simulink model "cm_test"  (R2015a)
settings: Solver=ode45  StartTime=0.0  StopTime=inf  MaxStep=1e-3  RelTol=1e-3
values from neighbouring files (symbols this model uses):
  ctr_law = struct    [Parameters.m]
  IMU = struct    [Parameters.m]
  lateral_control = true    [Parameters.m]
  longit_control = true    [Parameters.m]
  low_ctr = struct    [Parameters.m]
  mag = struct    [Parameters.m]
  steer_flag = 0    [Parameters.m]
  steer_sensor = struct    [Parameters.m]
  vhcl = struct    [Parameters.m]
undefined symbols (not defined in the file or in its folder): odo
libraries: CarMaker4SL x29, dspquant2 x6, simulink x1, aerolibtransform2 x1
(part 1 of 2)
settings Model: ExtModeAutoUpdateStatusClock=off  Creator=fh  LastModifiedBy=Robot
settings DataIOCC: SignalLoggingSaveFormat=ModelDataLogs  SignalLoggingName=sigsOut
settings OptimizationCC: BooleanDataType=off  ExpressionDepthLimit=2147483647  InitFltsAndDblsToZero=on
settings DebuggingCC: SaveWithParameterizedLinksMsg=none  SignalResolutionControl=TryResolveAllWithWarning  MultiTaskDSMMsg=warning  MultiTaskCondExecSysMsg=none  StateNameClashWarn=warning
settings HardwareCC: TargetUnknown=on
settings CodeAppCC: MaxIdLength=63
settings GRTTargetCC: TargetFcnLib=ansi_tfl_tmw.mat  CombineOutputUpdateFcns=off  GRTInterface=on
settings ConfigComp: CovMetricSettings=dw  CovHtmlReporting=on  CovSaveCumulativeToWorkspaceVar=on  CovSaveSingleToWorkspaceVar=on  CovExternalEMLEnable=off  CovSFcnEnable=off

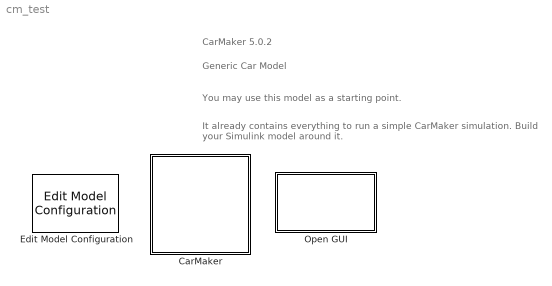
== system cm_test ==
  note: Generic Car Model
  note: You may use this model as a starting point.
  note: It already contains everything to run a simple CarMaker simulation.
      | Build your Simulink model around it.
  note: CarMaker 5.0.2
  CarMaker : Subsystem  TreatAsAtomicUnit=on
      mask Display: image(imread('CarMaker4SLss.bmp'));
  Edit Model Configuration : CarMaker4SL/Edit Model Configuration
  Open GUI : Subsystem  LoadFcn=if ~length(which('cmcmd')), cmenv; end
      settings: OpenFcn=cmblockmagic('gui_fix_display'); CM_Simulink
      mask Display: image(imread('CarMakerGUI.bmp'));

== system cm_test/CarMaker ==
  CM_FIRST : Subsystem
  CM_LAST : Subsystem
  DrivMan : Subsystem
  Ground : Ground
  IPG Vehicle : Subsystem  TreatAsAtomicUnit=on
  Terminator : Terminator
  VehicleControl : Subsystem
  wires:
  DrivMan/2(DrivMan.Out) -> VehicleControl/2(DrivMan.In)
  DrivMan/1(Sync_Out) -> VehicleControl/1(Sync_In)
  CM_FIRST/2(Env.Misc) -> DrivMan/2(Env.Misc)
  CM_FIRST/1(Sync_Out) -> DrivMan/1(Sync_In)
  CM_LAST/1(Sync_Out) -> Terminator/1
  IPG Vehicle/1(Sync_Out) -> CM_LAST/1(Sync_In)
  VehicleControl/1(Sync_Out) -> IPG Vehicle/1(Sync_In)
  VehicleControl/3(VhclCtrl.Steering) -> IPG Vehicle/3(VhclCtrl.Steering)
  VehicleControl/4(Vhcl.Wheel.In) -> IPG Vehicle/4(Vhcl.Wheel.In)
  VehicleControl/5(Vhcl.Misc) -> IPG Vehicle/5(Vhcl.Misc)
  VehicleControl/6(VhclCtrl.Brake) -> IPG Vehicle/6(VhclCtrl.Brake)
  VehicleControl/7(VhclCtrl.PT) -> IPG Vehicle/7(VhclCtrl.PT)
  VehicleControl/2(Vhcl.Model.Source) -> IPG Vehicle/2(Vhcl.Model.Source)
  Ground/1 -> CM_FIRST/1(Sync_In)

== system cm_test/Open GUI ==
  S-Function : S-Function  FunctionName=cm_gui

== system cm_test/CarMaker/CM_FIRST ==
  Sync_In : Inport
  Bus Creator1 : BusCreator  Inputs=9
  Demux : Demux  Outputs=9
  Environment : S-Function  FunctionName=CM_Sfun  Parameters='Environment'
  IoIn : S-Function  FunctionName=CM_Sfun  Parameters='IoIn'
  Sync_Out : Outport
  Env.Misc : Outport  Port=2
  wires:
  Bus Creator1/1 -> Env.Misc/1
  Environment/2 -> Demux/1
  Demux/4 -> Bus Creator1/4  "Env AirHumidity"
  Demux/3 -> Bus Creator1/3  "Env AirPressure"
  Demux/2 -> Bus Creator1/2  "Env AirDensity"
  Demux/1 -> Bus Creator1/1  "Env Temperature"
  Environment/1 -> Sync_Out/1
  IoIn/1 -> Environment/1
  Sync_In/1 -> IoIn/1
  Demux/5 -> Bus Creator1/5  "Env Time"
  Demux/6 -> Bus Creator1/6  "Env SolarRadiation"
  Demux/7 -> Bus Creator1/7  "Env WindVel_tot x"
  Demux/8 -> Bus Creator1/8  "Env WindVel_tot y"
  Demux/9 -> Bus Creator1/9  "Env WindVel_tot z"

== system cm_test/CarMaker/CM_LAST ==
  Sync_In : Inport
  CM_User : S-Function  FunctionName=CM_Sfun  Parameters='CM_User'
  IoOut : S-Function  FunctionName=CM_Sfun  Parameters='IoOut'
  Sync_Out : Outport
  wires:
  IoOut/1 -> Sync_Out/1
  CM_User/1 -> IoOut/1
  Sync_In/1 -> CM_User/1

== system cm_test/CarMaker/DrivMan ==
  note: There's rarely a reason to override DrivMan signals.
      | Use the VehicleControl interface for this purpose.
  Sync_In : Inport
  Env.Misc : Inport  Port=2
  BusCreator : BusCreator  Inputs=17
  Demux : Demux  Outputs=17
  DrivMan : S-Function  FunctionName=CM_Sfun  Parameters='DrivMan'
  Sync_Out : Outport
  DrivMan.Out : Outport  Port=2
  wires:
  Demux/17 -> BusCreator/17  "DrivMan Steering Trq"
  Demux/16 -> BusCreator/16  "DrivMan Steering AngAcc"
  Demux/15 -> BusCreator/15  "DrivMan Steering AngVel"
  Demux/14 -> BusCreator/14  "DrivMan Steering Ang"
  Demux/13 -> BusCreator/13  "DrivMan Gas"
  Demux/12 -> BusCreator/12  "DrivMan Clutch"
  Demux/11 -> BusCreator/11  "DrivMan BrakePark"
  Demux/10 -> BusCreator/10  "DrivMan Brake"
  Demux/9 -> BusCreator/9  "DrivMan GearNo"
  Demux/8 -> BusCreator/8  "DrivMan SelectorCtrl"
  Demux/7 -> BusCreator/7  "DrivMan UserSignal4"
  Demux/6 -> BusCreator/6  "DrivMan UserSignal3"
  Demux/5 -> BusCreator/5  "DrivMan UserSignal2"
  Demux/4 -> BusCreator/4  "DrivMan UserSignal1"
  Demux/3 -> BusCreator/3  "DrivMan UserSignal0"
  Demux/2 -> BusCreator/2  "DrivMan Key"
  Demux/1 -> BusCreator/1  "DrivMan SST"
  Env.Misc/1 -> DrivMan/2
  Sync_In/1 -> DrivMan/1
  DrivMan/1 -> Sync_Out/1
  BusCreator/1 -> DrivMan.Out/1
  DrivMan/2 -> Demux/1

== system cm_test/CarMaker/IPG Vehicle ==
  Sync_In : Inport
  Vhcl.Model.Source : Inport  Port=2
  VhclCtrl.Steering : Inport  Port=3
  Vhcl.Wheel.In : Inport  Port=4
  Vhcl.Misc : Inport  Port=5
  VhclCtrl.Brake : Inport  Port=6
  VhclCtrl.PT : Inport  Port=7
  Brake : Subsystem
  CarAndTrailer : Subsystem
  PowerTrain : Subsystem
  Stop Simulation : Stop
  VehicleSource_BuiltIn : simulink/Logic and Bit Operations/Compare To Constant  relop=~=  const=1  OutDataTypeStr=boolean  ZeroCross=off
  Sync_Out : Outport
  wires:
  VhclCtrl.PT/1 -> PowerTrain/3(VhclCtrl.PT)
  Brake/1(Sync_Out) -> PowerTrain/1(Sync_In)
  CarAndTrailer/1(Sync_Out) -> Brake/1(Sync_In)
  CarAndTrailer/2(Brake.IF.In) -> Brake/2(Brake.IF.In)
  VhclCtrl.Brake/1 -> Brake/3(VhclCtrl.Brake)
  PowerTrain/1(Sync_Out) -> Sync_Out/1
  Vhcl.Misc/1 -> CarAndTrailer/4(Vhcl.Misc)
  Vhcl.Wheel.In/1 -> CarAndTrailer/3(Vhcl.Wheel.In)
  VhclCtrl.Steering/1 -> CarAndTrailer/2(VhclCtrl.Steering)
  Sync_In/1 -> CarAndTrailer/1(Sync_In)
  Vhcl.Model.Source/1 -> VehicleSource_BuiltIn/1
  VehicleSource_BuiltIn/1 -> Stop Simulation/1
  Brake/2(Vhcl.Wheel.PT) -> PowerTrain/2(Vhcl.Wheel.PT)

== system cm_test/CarMaker/VehicleControl ==
  note: When implementing a vehicle control model,
      | be sure to add '-disablevehiclecontrol' to the command line arguments
      | in the CarMaker Model Configuration block.
      | Otherwise your model will possibly not see the original DrivMan signals
      | on its inputs, but those of a currently activated C-coded vehicle control model instead.
  Sync_In : Inport
  DrivMan.In : Inport  Port=2
  Autonomous driving : Subsystem
  Bus Creator2 : BusCreator  Inputs=2
  CreateBus Vhcl.Misc : Subsystem
  CreateBus Vhcl.Wheel.In : Subsystem
  CreateBus VhclCtrl : Subsystem
  CreateBus VhclCtrl.PT : Subsystem
  CreateBus VhclCtrl.Steering : Subsystem
  Demux2 : Demux  Outputs=2
  Sensors : Subsystem
  VehicleControl : S-Function  FunctionName=CM_Sfun  Parameters='VehicleControl'
  VehicleControlUpd : S-Function  FunctionName=CM_Sfun  Parameters='VehicleControlUpd'
  Sync_Out : Outport
  Vhcl.Model.Source : Outport  Port=2
  VhclCtrl.Steering : Outport  Port=3
  Vhcl.Wheel.In : Outport  Port=4
  Vhcl.Misc : Outport  Port=5
  VhclCtrl.Brake : Outport  Port=6
  VhclCtrl.PT : Outport  Port=7
  wires:
  VehicleControl/2 -> CreateBus VhclCtrl/1(Driver_In)
  VehicleControlUpd/2 -> Vhcl.Model.Source/1
  VehicleControlUpd/4 -> CreateBus Vhcl.Wheel.In/1(In1)
  VehicleControlUpd/5 -> CreateBus Vhcl.Misc/1(In1)
  VehicleControlUpd/6 -> Demux2/1
  VehicleControlUpd/7 -> CreateBus VhclCtrl.PT/1(In1)
  VehicleControlUpd/3 -> CreateBus VhclCtrl.Steering/1(In1)
  CreateBus Vhcl.Misc/1(Out1) -> Vhcl.Misc/1
  CreateBus Vhcl.Wheel.In/1(Out1) -> Vhcl.Wheel.In/1
  DrivMan.In/1 -> VehicleControl/2
  VehicleControl/1 -> VehicleControlUpd/1
  Sync_In/1 -> VehicleControl/1
  CreateBus VhclCtrl.PT/1(Out1) -> VhclCtrl.PT/1
  Bus Creator2/1 -> VhclCtrl.Brake/1
  CreateBus VhclCtrl.Steering/1(Out1) -> VhclCtrl.Steering/1
  VehicleControlUpd/1 -> Sync_Out/1
  Demux2/2 -> Bus Creator2/2  "VhclCtrl BrakePark"
  Demux2/1 -> Bus Creator2/1  "VhclCtrl Brake"
  Sensors/1(sensors_bus_out) -> Autonomous driving/1(sensors_in)
  CreateBus VhclCtrl/1(Out) -> VehicleControlUpd/2
  Autonomous driving/1(accel_ctrl_vars) -> CreateBus VhclCtrl/2(accel_ctrl_vars)
  Autonomous driving/2(steer_ctrl_vars) -> CreateBus VhclCtrl/3(steer_ctrl_vars)

== system cm_test/CarMaker/IPG Vehicle/Brake ==
  note: <Your model here>
  note: When replacing the entire braking system,
      | be sure to add '-disablebrake' to the command line arguments
      | in the CarMaker Model Configuration block.
  Sync_In : Inport
  Brake.IF.In : Inport  Port=2
  VhclCtrl.Brake : Inport  Port=3
  Brake : S-Function  FunctionName=CM_Sfun  Parameters='Brake'
  BrakeUpd : S-Function  FunctionName=CM_Sfun  Parameters='BrakeUpd'
  BusCreator : BusCreator  Inputs=12
  CreateBus Vhcl.Wheel.PT : Subsystem
  Demux : Demux  Outputs=12
  Sync_Out : Outport
  Vhcl.Wheel.PT : Outport  Port=2
  wires:
  BrakeUpd/1 -> Sync_Out/1
  Brake/1 -> BrakeUpd/1  "Sync"
  Brake.IF.In/1 -> Brake/2
  VhclCtrl.Brake/1 -> Brake/3
  Brake/2 -> Demux/1
  BusCreator/1 -> BrakeUpd/2
  Sync_In/1 -> Brake/1
  Demux/12 -> BusCreator/12  "Brake IF Trq_Reg_trg RR"
  Demux/11 -> BusCreator/11  "Brake IF Trq_Reg_trg RL"
  Demux/10 -> BusCreator/10  "Brake IF Trq_Reg_trg FR"
  Demux/9 -> BusCreator/9  "Brake IF Trq_Reg_trg FL"
  Demux/8 -> BusCreator/8  "Brake IF Trq_PB RR"
  Demux/7 -> BusCreator/7  "Brake IF Trq_PB RL"
  Demux/6 -> BusCreator/6  "Brake IF Trq_PB FR"
  Demux/5 -> BusCreator/5  "Brake IF Trq_PB FL"
  Demux/4 -> BusCreator/4  "Brake IF Trq_WB RR"
  Demux/3 -> BusCreator/3  "Brake IF Trq_WB RL"
  Demux/2 -> BusCreator/2  "Brake IF Trq_WB FR"
  Demux/1 -> BusCreator/1  "Brake IF Trq_WB FL"
  BrakeUpd/2 -> CreateBus Vhcl.Wheel.PT/1(In)
  CreateBus Vhcl.Wheel.PT/1(Out) -> Vhcl.Wheel.PT/1

== system cm_test/CarMaker/IPG Vehicle/CarAndTrailer ==
  Sync_In : Inport
  VhclCtrl.Steering : Inport  Port=2
  Vhcl.Wheel.In : Inport  Port=3
  Vhcl.Misc : Inport  Port=4
  CarAndTrailerUpd : Subsystem
  Forces : Subsystem
  Ground : Ground
  Kinematics : Subsystem
  Kinetics : Subsystem
  Steering : Subsystem
  Terminator : Terminator
  Terminator1 : Terminator
  Trailer : Subsystem
  Sync_Out : Outport
  Brake.IF.In : Outport  Port=2
  wires:
  Trailer/9(Car.Hitch.FrcTrq) -> CarAndTrailerUpd/9(Car.Hitch.FrcTrq)
  Trailer/8(Vhcl.Wheel.RR) -> CarAndTrailerUpd/8(Vhcl.Wheel.RR)
  Trailer/7(Vhcl.Wheel.RL) -> CarAndTrailerUpd/7(Vhcl.Wheel.RL)
  Trailer/6(Vhcl.Wheel.FR) -> CarAndTrailerUpd/6(Vhcl.Wheel.FR)
  Trailer/5(Vhcl.Wheel.FL) -> CarAndTrailerUpd/5(Vhcl.Wheel.FL)
  Trailer/4(Vhcl.PoI) -> CarAndTrailerUpd/4(Vhcl.PoI)
  Trailer/3(Vhcl.Motion) -> CarAndTrailerUpd/3(Vhcl.Motion)
  Trailer/2(Vhcl.Steering) -> CarAndTrailerUpd/2(Vhcl.Steering)
  Trailer/1(Sync_Out) -> CarAndTrailerUpd/1(Sync_In)
  CarAndTrailerUpd/2(Brake.IF.In) -> Brake.IF.In/1
  CarAndTrailerUpd/1(Sync_Out) -> Sync_Out/1
  Vhcl.Misc/1 -> Terminator1/1
  Vhcl.Wheel.In/1 -> Terminator/1
  Kinetics/6(WheelCarrier.Misc) -> Trailer/6(WheelCarrier.Misc)
  Kinetics/5(Car.Trq_T2W) -> Trailer/5(Car.Trq_T2W)
  Steering/2(Steer.IF) -> Kinematics/2(Steer.IF)
  Kinetics/4(Car.Fr1) -> Trailer/4(Car.Fr1)
  Kinetics/3(Car.Hitch) -> Trailer/3(Car.Hitch)
  Kinetics/2(Trailer.Load) -> Trailer/2(Trailer.Load)
  VhclCtrl.Steering/1 -> Steering/2(VhclCtrl.Steering)
  Sync_In/1 -> Steering/1(Sync_In)
  Steering/1(Sync_Out) -> Kinematics/1(Sync_In)
  Kinetics/1(Sync_Out) -> Trailer/1(Sync_In)
  Ground/1 -> CarAndTrailerUpd/10(Vhcl.Fr1A)
  Forces/11(FStabi) -> Kinetics/11(FStabi)
  Forces/10(FDamp) -> Kinetics/10(FDamp)
  Forces/9(FSpring) -> Kinetics/9(FSpring)
  Forces/8(TireRR_Out) -> Kinetics/8(TireRR.Out)
  Forces/7(TireRL_Out) -> Kinetics/7(TireRL.Out)
  Forces/6(TireFR_Out) -> Kinetics/6(TireFR.Out)
  Forces/5(TireFL_Out) -> Kinetics/5(TireFL.Out)
  Forces/4(Car.Load) -> Kinetics/4(Car.Load)
  Forces/2(Car.Virtual) -> Kinetics/2(Car.Virtual)
  Kinematics/6(lSpring) -> Forces/6(lSpring)
  Kinematics/7(vDamp) -> Forces/7(vDamp)
  Forces/3(Car.Aero) -> Kinetics/3(Car.Aero)
  Forces/1(Sync_Out) -> Kinetics/1(Sync_In)
  Kinematics/5(TireRR_In) -> Forces/5(TireRR_In)
  Kinematics/4(TireRL_In) -> Forces/4(TireRL_In)
  Kinematics/3(TireFR_In) -> Forces/3(TireFR_In)
  Kinematics/2(TireFL_In) -> Forces/2(TireFL_In)
  Kinematics/1(Sync_Out) -> Forces/1(Sync_In)
  Kinematics/8(lStabi) -> Forces/8(lStabi)
  Forces/12(FBuf) -> Kinetics/12(FBuf)
  Kinematics/9(lBuf) -> Forces/9(lBuf)

== system cm_test/CarMaker/IPG Vehicle/PowerTrain ==
  note: When replacing the entire powertrain,
      | be sure to add '-disablepowertrain' to the command line arguments
      | in the CarMaker Model Configuration block.
  note: <Your model here>
  Sync_In : Inport
  Vhcl.Wheel.PT : Inport  Port=2
  VhclCtrl.PT : Inport  Port=3
  BusCreator : BusCreator  Inputs=40
  Demux : Demux  Outputs=40
  PowerTrain : S-Function  FunctionName=CM_Sfun  Parameters='PowerTrain'
  PowerTrainUpd : S-Function  FunctionName=CM_Sfun  Parameters='PowerTrainUpd'
  Sync_Out : Outport
  wires:
  Sync_In/1 -> PowerTrain/1
  PowerTrain/2 -> Demux/1
  PowerTrainUpd/1 -> Sync_Out/1
  PowerTrain/1 -> PowerTrainUpd/1  "Sync"
  BusCreator/1 -> PowerTrainUpd/2
  Demux/1 -> BusCreator/1  "PT IF Ignition"
  Demux/2 -> BusCreator/2  "PT IF OperationState"
  Demux/3 -> BusCreator/3  "PT IF OperationError"
  Demux/4 -> BusCreator/4  "PT IF GearNo"
  Demux/5 -> BusCreator/5  "PT IF Engine_rotv"
  Demux/6 -> BusCreator/6  "PT IF Engine_Trq (EngineControl)"
  Demux/7 -> BusCreator/7  "PT IF Trq_Supp2Bdy1 x"
  Demux/8 -> BusCreator/8  "PT IF Trq_Supp2Bdy1 y"
  Demux/9 -> BusCreator/9  "PT IF Trq_Supp2Bdy1 z"
  Demux/10 -> BusCreator/10  "PT IF Trq_Supp2BdyEng x"
  Demux/11 -> BusCreator/11  "PT IF Trq_Supp2BdyEng y"
  Demux/12 -> BusCreator/12  "PT IF DL_iDiff_mean"
  Demux/13 -> BusCreator/13  "PT IF WFL rot"
  Demux/14 -> BusCreator/14  "PT IF WFL rotv"
  Demux/15 -> BusCreator/15  "PT IF WFL Trq_B2W"
  Demux/16 -> BusCreator/16  "PT IF WFL Trq_Drive"
  Demux/17 -> BusCreator/17  "PT IF WFL Trq_Supp2WC"
  Demux/18 -> BusCreator/18  "PT IF WFL Trq_BrakeReg"
  Demux/19 -> BusCreator/19  "PT IF WFL Trq_BrakeReg_max"
  Demux/20 -> BusCreator/20  "PT IF WFR rot"
  Demux/21 -> BusCreator/21  "PT IF WFR rotv"
  Demux/22 -> BusCreator/22  "PT IF WFR Trq_B2W"
  Demux/23 -> BusCreator/23  "PT IF WFR Trq_Drive"
  Demux/24 -> BusCreator/24  "PT IF WFR Trq_Supp2WC"
  Demux/25 -> BusCreator/25  "PT IF WFR Trq_BrakeReg"
  Demux/26 -> BusCreator/26  "PT IF WFR Trq_BrakeReg_max"
  Demux/27 -> BusCreator/27  "PT IF WRL rot"
  Demux/28 -> BusCreator/28  "PT IF WRL rotv"
  Demux/29 -> BusCreator/29  "PT IF WRL Trq_B2W"
  Demux/30 -> BusCreator/30  "PT IF WRL Trq_Drive"
  Demux/31 -> BusCreator/31  "PT IF WRL Trq_Supp2WC"
  Demux/32 -> BusCreator/32  "PT IF WRL Trq_BrakeReg"
  Demux/33 -> BusCreator/33  "PT IF WRL Trq_BrakeReg_max"
  Demux/34 -> BusCreator/34  "PT IF WRR rot"
  Demux/35 -> BusCreator/35  "PT IF WRR rotv"
  Demux/36 -> BusCreator/36  "PT IF WRR Trq_B2W"
  Demux/37 -> BusCreator/37  "PT IF WRR Trq_Drive"
  Demux/38 -> BusCreator/38  "PT IF WRR Trq_Supp2WC"
  Demux/39 -> BusCreator/39  "PT IF WRR Trq_BrakeReg"
  Demux/40 -> BusCreator/40  "PT IF WRR Trq_BrakeReg_max"
  VhclCtrl.PT/1 -> PowerTrain/3
  Vhcl.Wheel.PT/1 -> PowerTrain/2

== system cm_test/CarMaker/VehicleControl/Autonomous driving ==
  sensors_in : Inport
  Scope2 : Scope
      settings: YMin=-6  YMax=-3.25  SaveName=ScopeData17
  Selector : Selector  InputPortWidth=4  Indices=[1]
  ctr vars : Scope
      settings: ShowLegends=on  TimeRange=10  YMin=-1  YMax=9  SaveName=ScopeData8
  ctr_law structure : Constant  Value=ctr_law  OutDataTypeStr=Bus: ctr_law_params_bus
  low level control law structure def : Constant  Value=low_ctr  OutDataTypeStr=Bus: low_ctr_params_bus
  low level controller : MATLAB Function  TreatAsAtomicUnit=on  SystemSampleTime=1/low_ctr.Fs
  mem : Subsystem
  steer flag : Constant  Value=steer_flag
  steer ref : Scope
      settings: YMin=-0.75  YMax=0.75  SaveName=ScopeData13
  steering wheel angle : Scope
      settings: YMin=-6  YMax=-3.25  SaveName=ScopeData21
  trajectory tracking controller : MATLAB Function  TreatAsAtomicUnit=on  SystemSampleTime=1/ctr_law.Fs
  v_ref : Scope
      settings: YMin=1  YMax=12  SaveName=ScopeData2
  vhcl structure : Constant  Value=vhcl  OutDataTypeStr=Bus: vhcl_bus
  vhcl structure_bis : Constant  Value=vhcl  OutDataTypeStr=Bus: vhcl_bus
  accel_ctrl_vars : Outport  PortDimensions=2
  steer_ctrl_vars : Outport  Port=2
  wires:
  trajectory tracking controller/1(v) -> low level controller/2(v_ref), v_ref/1  "v_ref"
  sensors_in/1 -> low level controller/1(sensors_in), mem/1(sensors_in)
  ctr_law structure/1 -> trajectory tracking controller/2(ctr_law)
  vhcl structure/1 -> trajectory tracking controller/3(vehicle)
  trajectory tracking controller/2(gamma) -> low level controller/3(gamma_ref), steer ref/1  "gamma_ref"
  steer flag/1 -> low level controller/4(steer_flag)
  low level controller/1(accel) -> Scope2/1, accel_ctrl_vars/1
  low level control law structure def/1 -> low level controller/5(low_ctr)
  vhcl structure_bis/1 -> low level controller/6(vhcl)
  low level controller/2(steer) -> Selector/1, steer_ctrl_vars/1
  Selector/1 -> steering wheel angle/1
  trajectory tracking controller/3(ctr_vars) -> ctr vars/1
  mem/1(sensors_buffer) -> trajectory tracking controller/1(sensors_in)

== system cm_test/CarMaker/VehicleControl/CreateBus Vhcl.Misc ==
  In1 : Inport
  Bus Creator5 : BusCreator  Inputs=11
  Demux5 : Demux  Outputs=11
  Out1 : Outport
  wires:
  Demux5/11 -> Bus Creator5/11  "Vhcl Wind_vel_0 z"
  Demux5/10 -> Bus Creator5/10  "Vhcl Wind_vel_0 y"
  Demux5/9 -> Bus Creator5/9  "Vhcl Wind_vel_0 x"
  Demux5/8 -> Bus Creator5/8  "Vhcl DL2BdyEng y"
  Demux5/7 -> Bus Creator5/7  "Vhcl DL2BdyEng x"
  Demux5/6 -> Bus Creator5/6  "Vhcl TrqDL2Bdy1B z"
  Demux5/5 -> Bus Creator5/5  "Vhcl TrqDL2Bdy1B y"
  Demux5/4 -> Bus Creator5/4  "Vhcl TrqDL2Bdy1B x"
  Demux5/3 -> Bus Creator5/3  "Vhcl Trq_DL2Bdy1 z"
  In1/1 -> Demux5/1
  Bus Creator5/1 -> Out1/1
  Demux5/2 -> Bus Creator5/2  "Vhcl Trq_DL2Bdy1 y"
  Demux5/1 -> Bus Creator5/1  "Vhcl Trq_DL2Bdy1 x"

== system cm_test/CarMaker/VehicleControl/CreateBus Vhcl.Wheel.In ==
  In1 : Inport
  Bus Creator1 : BusCreator  Inputs=12
  Demux1 : Demux  Outputs=12
  Out1 : Outport
  wires:
  Demux1/12 -> Bus Creator1/12  "Vhcl Wheel RR rotv"
  Demux1/11 -> Bus Creator1/11  "Vhcl Wheel RR Trq_DL2WC"
  Demux1/10 -> Bus Creator1/10  "Vhcl Wheel RR Trq_B2WC"
  Demux1/9 -> Bus Creator1/9  "Vhcl Wheel RL rotv"
  Demux1/8 -> Bus Creator1/8  "Vhcl Wheel RL Trq_DL2WC"
  Demux1/7 -> Bus Creator1/7  "Vhcl Wheel RL Trq_B2WC"
  Demux1/6 -> Bus Creator1/6  "Vhcl Wheel FR rotv"
  Demux1/5 -> Bus Creator1/5  "Vhcl Wheel FR Trq_DL2WC"
  Demux1/4 -> Bus Creator1/4  "Vhcl Wheel FR Trq_B2WC"
  Demux1/3 -> Bus Creator1/3  "Vhcl Wheel FL rotv"
  In1/1 -> Demux1/1
  Bus Creator1/1 -> Out1/1
  Demux1/2 -> Bus Creator1/2  "Vhcl Wheel FL Trq_DL2WC"
  Demux1/1 -> Bus Creator1/1  "Vhcl Wheel FL Trq_B2WC"

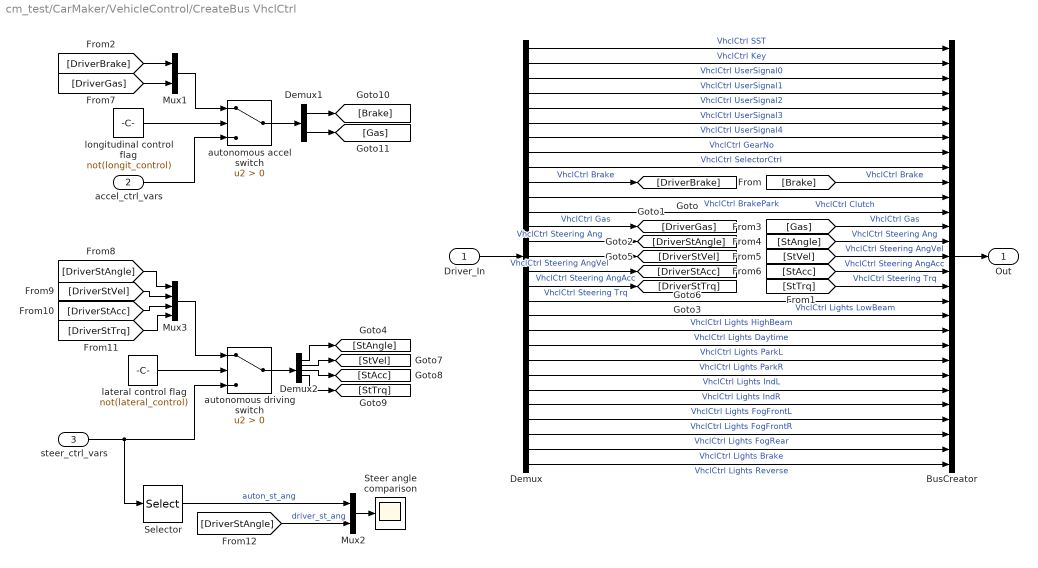
== system cm_test/CarMaker/VehicleControl/CreateBus VhclCtrl ==
  Driver_In : Inport
  accel_ctrl_vars : Inport  Port=2  PortDimensions=2
  steer_ctrl_vars : Inport  Port=3
  BusCreator : BusCreator  Inputs=29
  Demux : Demux  Outputs=29
  Demux1 : Demux  Outputs=2
  Demux2 : Demux
  Mux1 : Mux  Inputs=2
  Mux2 : Mux  Inputs=2
  Mux3 : Mux
  Selector : Selector  InputPortWidth=4  Indices=[1]
  Steer angle comparison : Scope
      settings: ShowLegends=on  YMin=-12.5  YMax=7.5  SaveName=ScopeData6
  autonomous accel switch : Switch  Criteria=u2 > Threshold
  autonomous driving switch : Switch  Criteria=u2 > Threshold
  lateral control flag : Constant  Value=not(lateral_control)
  longitudinal control flag : Constant  Value=not(longit_control)
  Out : Outport
  wires:
  Driver_In/1 -> Demux/1
  BusCreator/1 -> Out/1
  Demux/1 -> BusCreator/1  "VhclCtrl SST"
  Demux/2 -> BusCreator/2  "VhclCtrl Key"
  Demux/3 -> BusCreator/3  "VhclCtrl UserSignal0"
  Demux/4 -> BusCreator/4  "VhclCtrl UserSignal1"
  Demux/5 -> BusCreator/5  "VhclCtrl UserSignal2"
  Demux/6 -> BusCreator/6  "VhclCtrl UserSignal3"
  Demux/7 -> BusCreator/7  "VhclCtrl UserSignal4"
  Demux/8 -> BusCreator/8  "VhclCtrl GearNo"
  Demux/9 -> BusCreator/9  "VhclCtrl SelectorCtrl"
  Demux/11 -> BusCreator/11  "VhclCtrl BrakePark"
  Demux/12 -> BusCreator/12  "VhclCtrl Clutch"
  Demux/18 -> BusCreator/18  "VhclCtrl Lights LowBeam"
  Demux/19 -> BusCreator/19  "VhclCtrl Lights HighBeam"
  Demux/20 -> BusCreator/20  "VhclCtrl Lights Daytime"
  Demux/21 -> BusCreator/21  "VhclCtrl Lights ParkL"
  Demux/22 -> BusCreator/22  "VhclCtrl Lights ParkR"
  Demux/23 -> BusCreator/23  "VhclCtrl Lights IndL"
  Demux/24 -> BusCreator/24  "VhclCtrl Lights IndR"
  Demux/25 -> BusCreator/25  "VhclCtrl Lights FogFrontL"
  Demux/26 -> BusCreator/26  "VhclCtrl Lights FogFrontR"
  Demux/27 -> BusCreator/27  "VhclCtrl Lights FogRear"
  Demux/28 -> BusCreator/28  "VhclCtrl Lights Brake"
  Demux/29 -> BusCreator/29  "VhclCtrl Lights Reverse"
  Demux/10 -> [DriverBrake]  "VhclCtrl Brake"
  [Brake] -> BusCreator/10  "VhclCtrl Brake"
  Demux/13 -> [DriverGas]  "VhclCtrl Gas"
  [Gas] -> BusCreator/13  "VhclCtrl Gas"
  Demux/14 -> [DriverStAngle]  "VhclCtrl Steering Ang"
  Demux/15 -> [DriverStVel]  "VhclCtrl Steering AngVel"
  [StAngle] -> BusCreator/14  "VhclCtrl Steering Ang"
  [StVel] -> BusCreator/15  "VhclCtrl Steering AngVel"
  Demux/16 -> [DriverStAcc]  "VhclCtrl Steering AngAcc"
  [StAcc] -> BusCreator/16  "VhclCtrl Steering AngAcc"
  Demux/17 -> [DriverStTrq]  "VhclCtrl Steering Trq"
  [StTrq] -> BusCreator/17  "VhclCtrl Steering Trq"
  [DriverBrake] -> Mux1/1
  [DriverGas] -> Mux1/2
  Mux1/1 -> autonomous accel switch/1
  autonomous accel switch/1 -> Demux1/1
  Mux3/1 -> autonomous driving switch/1
  steer_ctrl_vars/1 -> Selector/1, autonomous driving switch/3
  autonomous driving switch/1 -> Demux2/1
  [DriverStAngle] -> Mux3/1
  [DriverStVel] -> Mux3/2
  [DriverStAcc] -> Mux3/3
  [DriverStTrq] -> Mux3/4
  Demux2/1 -> [StAngle]
  Demux2/2 -> [StVel]
  Demux2/3 -> [StAcc]
  Demux2/4 -> [StTrq]
  Demux1/1 -> [Brake]
  Demux1/2 -> [Gas]
  accel_ctrl_vars/1 -> autonomous accel switch/3
  longitudinal control flag/1 -> autonomous accel switch/2
  lateral control flag/1 -> autonomous driving switch/2
  Selector/1 -> Mux2/1  "auton_st_ang"
  [DriverStAngle] -> Mux2/2  "driver_st_ang"
  Mux2/1 -> Steer angle comparison/1

== system cm_test/CarMaker/VehicleControl/CreateBus VhclCtrl.PT ==
  In1 : Inport
  BusCreator : BusCreator  Inputs=11
  Demux : Demux  Outputs=11
  Out1 : Outport
  wires:
  In1/1 -> Demux/1
  BusCreator/1 -> Out1/1
  Demux/1 -> BusCreator/1  "VhclCtrl SST"
  Demux/2 -> BusCreator/2  "VhclCtrl Key"
  Demux/3 -> BusCreator/3  "VhclCtrl UserSignal0"
  Demux/4 -> BusCreator/4  "VhclCtrl UserSignal1"
  Demux/5 -> BusCreator/5  "VhclCtrl UserSignal2"
  Demux/6 -> BusCreator/6  "VhclCtrl UserSignal3"
  Demux/7 -> BusCreator/7  "VhclCtrl UserSignal4"
  Demux/8 -> BusCreator/8  "VhclCtrl GearNo"
  Demux/9 -> BusCreator/9  "VhclCtrl SelectorCtrl"
  Demux/10 -> BusCreator/10  "VhclCtrl Clutch"
  Demux/11 -> BusCreator/11  "VhclCtrl Gas"

== system cm_test/CarMaker/VehicleControl/CreateBus VhclCtrl.Steering ==
  In1 : Inport
  Bus Creator : BusCreator  Inputs=5
  Demux : Demux  Outputs=5
  Out1 : Outport
  wires:
  In1/1 -> Demux/1
  Bus Creator/1 -> Out1/1
  Demux/1 -> Bus Creator/1  "VhclCtrl Steering Ang"
  Demux/5 -> Bus Creator/5  "VhclCtrl Steering ByTrq"
  Demux/3 -> Bus Creator/3  "VhclCtrl Steering AngAcc"
  Demux/2 -> Bus Creator/2  "VhclCtrl Steering AngVel"
  Demux/4 -> Bus Creator/4  "VhclCtrl Steering Trq"

== system cm_test/CarMaker/VehicleControl/Sensors ==
  Bus Creator : BusCreator  Inputs=5  OutDataTypeStr=Bus: SensorsOut_bus  NonVirtualBus=on
  IMU : Subsystem
  Magnetometer : Subsystem
  RPSensor : Subsystem
  Steering angle (rad) : Subsystem
  odometry : Subsystem
  sensors_bus_out : Outport
  wires:
  Steering angle (rad)/1(steer angles) -> Bus Creator/4  "steersensor_out"
  Bus Creator/1 -> sensors_bus_out/1
  IMU/1(imu_out) -> Bus Creator/1  "imu_out"
  RPSensor/1(road_props) -> Bus Creator/3  "rpsensor_out"
  Magnetometer/1(mag_out) -> Bus Creator/2  "mag_out"
  odometry/1(odo_out) -> Bus Creator/5  "odo_out"

== system cm_test/CarMaker/IPG Vehicle/Brake/CreateBus Vhcl.Wheel.PT ==
  In : Inport
  BusCreator : BusCreator  Inputs=16
  Demux : Demux  Outputs=16
  Out : Outport
  wires:
  Demux/16 -> BusCreator/16  "Vhcl Wheel RR WhlBearing"
  Demux/15 -> BusCreator/15  "Vhcl Wheel RR Trq_T2W"
  Demux/14 -> BusCreator/14  "Vhcl Wheel RR Trq_BrakeReg_trg"
  Demux/13 -> BusCreator/13  "Vhcl Wheel RR Trq_Brake"
  Demux/12 -> BusCreator/12  "Vhcl Wheel RL WhlBearing"
  Demux/11 -> BusCreator/11  "Vhcl Wheel RL Trq_T2W"
  Demux/10 -> BusCreator/10  "Vhcl Wheel RL Trq_BrakeReg_trg"
  Demux/9 -> BusCreator/9  "Vhcl Wheel RL Trq_Brake"
  Demux/8 -> BusCreator/8  "Vhcl Wheel FR WhlBearing"
  Demux/7 -> BusCreator/7  "Vhcl Wheel FR Trq_T2W"
  Demux/6 -> BusCreator/6  "Vhcl Wheel FR Trq_BrakeReg_trg"
  Demux/5 -> BusCreator/5  "Vhcl Wheel FR Trq_Brake"
  Demux/4 -> BusCreator/4  "Vhcl Wheel FL WhlBearing"
  Demux/3 -> BusCreator/3  "Vhcl Wheel FL Trq_T2W"
  Demux/2 -> BusCreator/2  "Vhcl Wheel FL Trq_BrakeReg_trg"
  Demux/1 -> BusCreator/1  "Vhcl Wheel FL Trq_Brake"
  BusCreator/1 -> Out/1
  In/1 -> Demux/1

== system cm_test/CarMaker/IPG Vehicle/CarAndTrailer/CarAndTrailerUpd ==
  Sync_In : Inport
  Vhcl.Steering : Inport  Port=2
  Vhcl.Motion : Inport  Port=3
  Vhcl.PoI : Inport  Port=4
  Vhcl.Wheel.FL : Inport  Port=5
  Vhcl.Wheel.FR : Inport  Port=6
  Vhcl.Wheel.RL : Inport  Port=7
  Vhcl.Wheel.RR : Inport  Port=8
  Car.Hitch.FrcTrq : Inport  Port=9
  Vhcl.Fr1A : Inport  Port=10
  CarAndTrailerUpd : S-Function  FunctionName=CM_Sfun  Parameters='CarAndTrUpd'
  CreateBus Brake.IF.In : Subsystem
  Sync_Out : Outport
  Brake.IF.In : Outport  Port=2
  wires:
  Vhcl.Fr1A/1 -> CarAndTrailerUpd/10  "user vehicle only"
  Vhcl.Steering/1 -> CarAndTrailerUpd/2
  Vhcl.Motion/1 -> CarAndTrailerUpd/3
  Vhcl.PoI/1 -> CarAndTrailerUpd/4
  Vhcl.Wheel.FL/1 -> CarAndTrailerUpd/5
  Vhcl.Wheel.FR/1 -> CarAndTrailerUpd/6
  Car.Hitch.FrcTrq/1 -> CarAndTrailerUpd/9
  Vhcl.Wheel.RR/1 -> CarAndTrailerUpd/8
  Vhcl.Wheel.RL/1 -> CarAndTrailerUpd/7
  CarAndTrailerUpd/2 -> CreateBus Brake.IF.In/1(In)
  CreateBus Brake.IF.In/1(Out) -> Brake.IF.In/1
  CarAndTrailerUpd/1 -> Sync_Out/1
  Sync_In/1 -> CarAndTrailerUpd/1

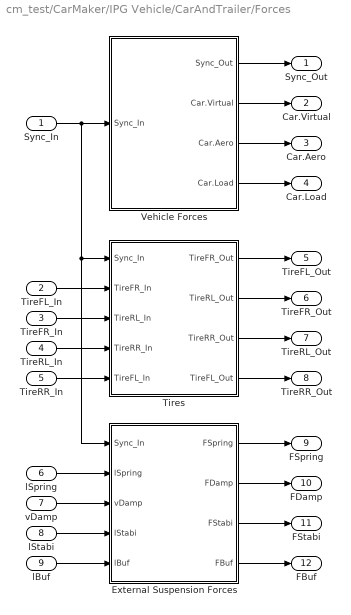
== system cm_test/CarMaker/IPG Vehicle/CarAndTrailer/Forces ==
  Sync_In : Inport
  TireFL_In : Inport  Port=2
  TireFR_In : Inport  Port=3
  TireRL_In : Inport  Port=4
  TireRR_In : Inport  Port=5
  lSpring : Inport  Port=6
  vDamp : Inport  Port=7
  lStabi : Inport  Port=8
  lBuf : Inport  Port=9
  External Suspension Forces : Subsystem
  Tires : Subsystem
  Vehicle Forces : Subsystem
  Sync_Out : Outport
  Car.Virtual : Outport  Port=2
  Car.Aero : Outport  Port=3
  Car.Load : Outport  Port=4
  TireFL_Out : Outport  Port=5
  TireFR_Out : Outport  Port=6
  TireRL_Out : Outport  Port=7
  TireRR_Out : Outport  Port=8
  FSpring : Outport  Port=9
  FDamp : Outport  Port=10
  FStabi : Outport  Port=11
  FBuf : Outport  Port=12
  wires:
  External Suspension Forces/4(FBuf) -> FBuf/1
  lBuf/1 -> External Suspension Forces/5(lBuf)
  Tires/4(TireFL_Out) -> TireRR_Out/1
  Tires/3(TireRR_Out) -> TireRL_Out/1
  Tires/2(TireRL_Out) -> TireFR_Out/1
  Tires/1(TireFR_Out) -> TireFL_Out/1
  TireRR_In/1 -> Tires/5(TireFL_In)
  TireRL_In/1 -> Tires/4(TireRR_In)
  TireFR_In/1 -> Tires/3(TireRL_In)
  Sync_In/1 -> External Suspension Forces/1(Sync_In), Tires/1(Sync_In), Vehicle Forces/1(Sync_In)
  Vehicle Forces/1(Sync_Out) -> Sync_Out/1
  TireFL_In/1 -> Tires/2(TireFR_In)
  Vehicle Forces/2(Car.Virtual) -> Car.Virtual/1
  Vehicle Forces/3(Car.Aero) -> Car.Aero/1
  Vehicle Forces/4(Car.Load) -> Car.Load/1
  lSpring/1 -> External Suspension Forces/2(lSpring)
  External Suspension Forces/2(FDamp) -> FDamp/1
  vDamp/1 -> External Suspension Forces/3(vDamp)
  lStabi/1 -> External Suspension Forces/4(lStabi)
  External Suspension Forces/3(FStabi) -> FStabi/1
  External Suspension Forces/1(FSpring) -> FSpring/1

== system cm_test/CarMaker/IPG Vehicle/CarAndTrailer/Kinematics ==
  Sync_In : Inport
  Steer.IF : Inport  Port=2
  Kinematics : S-Function  FunctionName=CM_Sfun  Parameters='Kinematics'
  Sync_Out : Outport
  TireFL_In : Outport  Port=2
  TireFR_In : Outport  Port=3
  TireRL_In : Outport  Port=4
  TireRR_In : Outport  Port=5
  lSpring : Outport  Port=6
  vDamp : Outport  Port=7
  lStabi : Outport  Port=8
  lBuf : Outport  Port=9
  wires:
  Kinematics/9 -> lBuf/1
  Kinematics/8 -> lStabi/1
  Kinematics/2 -> TireFL_In/1
  Kinematics/3 -> TireFR_In/1
  Kinematics/4 -> TireRL_In/1
  Kinematics/5 -> TireRR_In/1
  Kinematics/6 -> lSpring/1
  Kinematics/7 -> vDamp/1
  Sync_In/1 -> Kinematics/1
  Kinematics/1 -> Sync_Out/1
  Steer.IF/1 -> Kinematics/2

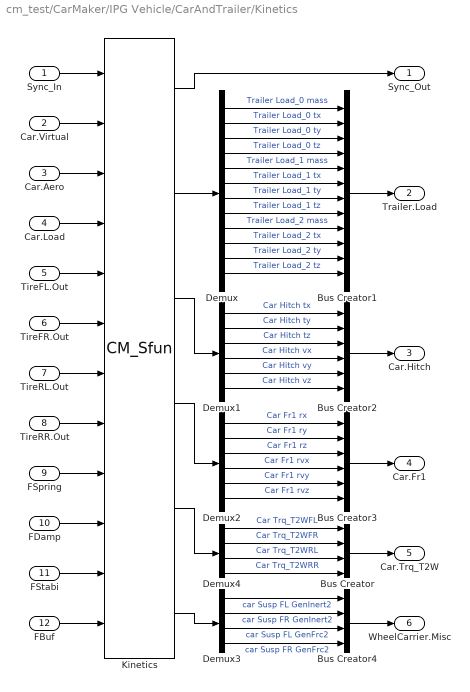
== system cm_test/CarMaker/IPG Vehicle/CarAndTrailer/Kinetics ==
  Sync_In : Inport
  Car.Virtual : Inport  Port=2
  Car.Aero : Inport  Port=3
  Car.Load : Inport  Port=4
  TireFL.Out : Inport  Port=5
  TireFR.Out : Inport  Port=6
  TireRL.Out : Inport  Port=7
  TireRR.Out : Inport  Port=8
  FSpring : Inport  Port=9
  FDamp : Inport  Port=10
  FStabi : Inport  Port=11
  FBuf : Inport  Port=12
  Bus Creator : BusCreator
  Bus Creator1 : BusCreator  Inputs=12
  Bus Creator2 : BusCreator  Inputs=6
  Bus Creator3 : BusCreator  Inputs=6
  Bus Creator4 : BusCreator
  Demux : Demux  Outputs=12
  Demux1 : Demux  Outputs=6
  Demux2 : Demux  Outputs=6
  Demux3 : Demux
  Demux4 : Demux
  Kinetics : S-Function  FunctionName=CM_Sfun  Parameters='Kinetics'
  Sync_Out : Outport
  Trailer.Load : Outport  Port=2
  Car.Hitch : Outport  Port=3
  Car.Fr1 : Outport  Port=4
  Car.Trq_T2W : Outport  Port=5
  WheelCarrier.Misc : Outport  Port=6
  wires:
  FBuf/1 -> Kinetics/12
  Sync_In/1 -> Kinetics/1
  Kinetics/1 -> Sync_Out/1
  Car.Aero/1 -> Kinetics/3
  Car.Virtual/1 -> Kinetics/2
  Bus Creator1/1 -> Trailer.Load/1
  Demux/1 -> Bus Creator1/1  "Trailer Load_0 mass"
  Demux/2 -> Bus Creator1/2  "Trailer Load_0 tx"
  Demux/3 -> Bus Creator1/3  "Trailer Load_0 ty"
  Demux/4 -> Bus Creator1/4  "Trailer Load_0 tz"
  Kinetics/2 -> Demux/1
  Demux/5 -> Bus Creator1/5  "Trailer Load_1 mass"
  Demux/6 -> Bus Creator1/6  "Trailer Load_1 tx"
  Demux/7 -> Bus Creator1/7  "Trailer Load_1 ty"
  Demux/8 -> Bus Creator1/8  "Trailer Load_1 tz"
  Demux/9 -> Bus Creator1/9  "Trailer Load_2 mass"
  Demux/10 -> Bus Creator1/10  "Trailer Load_2 tx"
  Demux/11 -> Bus Creator1/11  "Trailer Load_2 ty"
  Demux/12 -> Bus Creator1/12  "Trailer Load_2 tz"
  Demux1/1 -> Bus Creator2/1  "Car Hitch tx"
  Demux1/2 -> Bus Creator2/2  "Car Hitch ty"
  Demux1/3 -> Bus Creator2/3  "Car Hitch tz"
  Demux1/4 -> Bus Creator2/4  "Car Hitch vx"
  Demux1/5 -> Bus Creator2/5  "Car Hitch vy"
  Demux1/6 -> Bus Creator2/6  "Car Hitch vz"
  Kinetics/3 -> Demux1/1
  Bus Creator2/1 -> Car.Hitch/1
  Demux2/1 -> Bus Creator3/1  "Car Fr1 rx"
  Demux2/2 -> Bus Creator3/2  "Car Fr1 ry"
  Demux2/3 -> Bus Creator3/3  "Car Fr1 rz"
  Demux2/4 -> Bus Creator3/4  "Car Fr1 rvx"
  Demux2/5 -> Bus Creator3/5  "Car Fr1 rvy"
  Demux2/6 -> Bus Creator3/6  "Car Fr1 rvz"
  Bus Creator3/1 -> Car.Fr1/1
  Kinetics/4 -> Demux2/1
  Car.Load/1 -> Kinetics/4
  Demux3/1 -> Bus Creator4/1  "car Susp FL GenInert2"
  Demux3/2 -> Bus Creator4/2  "car Susp FR GenInert2"
  Demux3/3 -> Bus Creator4/3  "car Susp FL GenFrc2"
  Demux3/4 -> Bus Creator4/4  "car Susp FR GenFrc2"
  Bus Creator4/1 -> WheelCarrier.Misc/1
  Bus Creator/1 -> Car.Trq_T2W/1
  Demux4/4 -> Bus Creator/4  "Car Trq_T2WRR"
  Demux4/3 -> Bus Creator/3  "Car Trq_T2WRL"
  Demux4/2 -> Bus Creator/2  "Car Trq_T2WFR"
  Demux4/1 -> Bus Creator/1  "Car Trq_T2WFL"
  TireFL.Out/1 -> Kinetics/5
  TireFR.Out/1 -> Kinetics/6
  TireRL.Out/1 -> Kinetics/7
  TireRR.Out/1 -> Kinetics/8
  FSpring/1 -> Kinetics/9
  FDamp/1 -> Kinetics/10
  FStabi/1 -> Kinetics/11
  Kinetics/6 -> Demux3/1
  Kinetics/5 -> Demux4/1

== system cm_test/CarMaker/IPG Vehicle/CarAndTrailer/Steering ==
  note: When replacing the entire steering system,
      | be sure to add '-disablesteering' to the command line arguments
      | in the CarMaker Model Configuration block.
  Sync_In : Inport
  VhclCtrl.Steering : Inport  Port=2
  Bus Creator1 : BusCreator  Inputs=16
  Bus Creator2 : BusCreator
  Demux : Demux  Outputs=20
  Steering : S-Function  FunctionName=CM_Sfun  Parameters='Steering'
  Terminator : Terminator
  Sync_Out : Outport
  Steer.IF : Outport  Port=2
  wires:
  Bus Creator1/1 -> Steer.IF/1
  Steering/2 -> Demux/1
  Demux/8 -> Bus Creator1/8  "Steering IF AssistTrqPin"
  Demux/7 -> Bus Creator1/7  "Steering IF AssistTrqCol"
  Demux/6 -> Bus Creator1/6  "Steering IF AssistFrc"
  Demux/20 -> Bus Creator2/4  "Steering IF R Inert"
  Demux/17 -> Bus Creator2/1  "Steering IF L Frc"
  Demux/18 -> Bus Creator2/2  "Steering IF L Inert"
  Demux/19 -> Bus Creator2/3  "Steering IF R Frc"
  Bus Creator2/1 -> Terminator/1  "Steer IF (in)"
  Demux/16 -> Bus Creator1/16  "Steering IF R iSteer2q"
  Demux/9 -> Bus Creator1/9  "Steering IF L q"
  Demux/10 -> Bus Creator1/10  "Steering IF L qp"
  Demux/11 -> Bus Creator1/11  "Steering IF L qpp"
  Demux/12 -> Bus Creator1/12  "Steering IF L iSteer2q"
  Demux/13 -> Bus Creator1/13  "Steering IF R q"
  Demux/14 -> Bus Creator1/14  "Steering IF R qp"
  Demux/15 -> Bus Creator1/15  "Steering IF R qpp"
  VhclCtrl.Steering/1 -> Steering/2
  Steering/1 -> Sync_Out/1
  Sync_In/1 -> Steering/1
  Demux/1 -> Bus Creator1/1  "Steering IF Ang"
  Demux/2 -> Bus Creator1/2  "Steering IF AngVel"
  Demux/3 -> Bus Creator1/3  "Steering IF AngAcc"
  Demux/4 -> Bus Creator1/4  "Steering IF Trq"
  Demux/5 -> Bus Creator1/5  "Steering IF TrqStatic"

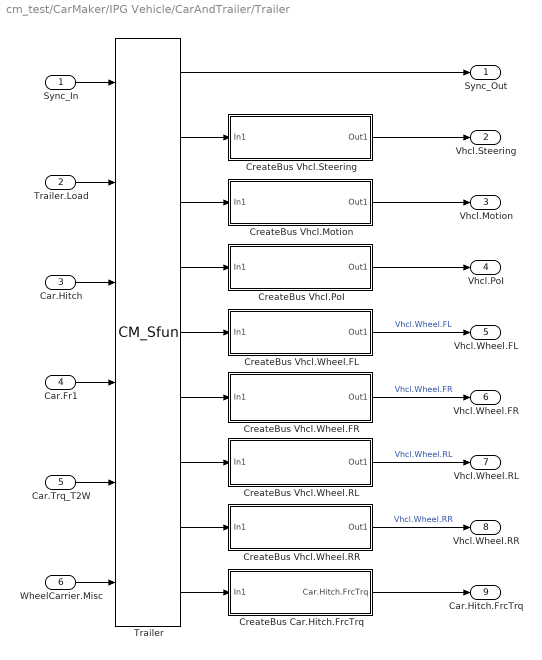
== system cm_test/CarMaker/IPG Vehicle/CarAndTrailer/Trailer ==
  Sync_In : Inport
  Trailer.Load : Inport  Port=2
  Car.Hitch : Inport  Port=3
  Car.Fr1 : Inport  Port=4
  Car.Trq_T2W : Inport  Port=5
  WheelCarrier.Misc : Inport  Port=6
  CreateBus Car.Hitch.FrcTrq : Subsystem
  CreateBus Vhcl.Motion : Subsystem
  CreateBus Vhcl.PoI : Subsystem
  CreateBus Vhcl.Steering : Subsystem
  CreateBus Vhcl.Wheel.FL : Subsystem
  CreateBus Vhcl.Wheel.FR : Subsystem
  CreateBus Vhcl.Wheel.RL : Subsystem
  CreateBus Vhcl.Wheel.RR : Subsystem
  Trailer : S-Function  FunctionName=CM_Sfun  Parameters='Trailer'
  Sync_Out : Outport
  Vhcl.Steering : Outport  Port=2
  Vhcl.Motion : Outport  Port=3
  Vhcl.PoI : Outport  Port=4
  Vhcl.Wheel.FL : Outport  Port=5
  Vhcl.Wheel.FR : Outport  Port=6
  Vhcl.Wheel.RL : Outport  Port=7
  Vhcl.Wheel.RR : Outport  Port=8
  Car.Hitch.FrcTrq : Outport  Port=9
  wires:
  Trailer/2 -> CreateBus Vhcl.Steering/1(In1)
  CreateBus Vhcl.Steering/1(Out1) -> Vhcl.Steering/1
  Trailer/3 -> CreateBus Vhcl.Motion/1(In1)
  Trailer/4 -> CreateBus Vhcl.PoI/1(In1)
  Trailer/5 -> CreateBus Vhcl.Wheel.FL/1(In1)
  Trailer/6 -> CreateBus Vhcl.Wheel.FR/1(In1)
  Trailer/7 -> CreateBus Vhcl.Wheel.RL/1(In1)
  Trailer/9 -> CreateBus Car.Hitch.FrcTrq/1(In1)
  Trailer/8 -> CreateBus Vhcl.Wheel.RR/1(In1)
  CreateBus Vhcl.Wheel.RR/1(Out1) -> Vhcl.Wheel.RR/1  "Vhcl.Wheel.RR"
  CreateBus Vhcl.Wheel.RL/1(Out1) -> Vhcl.Wheel.RL/1  "Vhcl.Wheel.RL"
  CreateBus Vhcl.Wheel.FR/1(Out1) -> Vhcl.Wheel.FR/1  "Vhcl.Wheel.FR"
  CreateBus Vhcl.Wheel.FL/1(Out1) -> Vhcl.Wheel.FL/1  "Vhcl.Wheel.FL"
  CreateBus Vhcl.PoI/1(Out1) -> Vhcl.PoI/1
  CreateBus Vhcl.Motion/1(Out1) -> Vhcl.Motion/1
  Car.Trq_T2W/1 -> Trailer/5
  WheelCarrier.Misc/1 -> Trailer/6
  CreateBus Car.Hitch.FrcTrq/1(Car.Hitch.FrcTrq) -> Car.Hitch.FrcTrq/1
  Car.Fr1/1 -> Trailer/4
  Car.Hitch/1 -> Trailer/3
  Trailer.Load/1 -> Trailer/2
  Trailer/1 -> Sync_Out/1
  Sync_In/1 -> Trailer/1

== system cm_test/CarMaker/VehicleControl/Autonomous driving/mem ==
  sensors_in : Inport
  Memory : Memory
  Memory1 : Memory
  Memory2 : Memory
  Vector Concatenate : Concatenate  NumInputs=4
  sensors_buffer : Outport
  wires:
  sensors_in/1 -> Vector Concatenate/1, Memory/1
  Memory/1 -> Vector Concatenate/2, Memory1/1
  Memory1/1 -> Vector Concatenate/3, Memory2/1
  Vector Concatenate/1 -> sensors_buffer/1
  Memory2/1 -> Vector Concatenate/4

== system cm_test/CarMaker/VehicleControl/Sensors/IMU ==
  Accelerometers : Subsystem
  Accels : Scope
      settings: SaveName=ScopeData7  Decimation=10
  Bus Creator : BusCreator  Inputs='Omega_0','Alpha_0'  OutDataTypeStr=Bus: imu_bus  NonVirtualBus=on
  Demux1 : Demux  Outputs=[3 3]
  Downsample : DownSample  N=IMU.K_dn
  Gyroscopes : Subsystem
  Mux : Mux  Inputs=2
  Scalar Quantizer Encoder : dspquant2/Scalar Quantizer Encoder  paramSrc=Specify via dialog  partType=Bounded  BBoundary=IMU.gyro.bnd_pts  UBoundary=[2:9]  SearchMethod=Linear  tieBreakRule=Choose the lower index  outQU=on  outQError=off  codebook=IMU.gyro.bnd_pts(1:end-1)  outStatus=off  invalidin=Clip  idtype=int32  roundingMode=Nearest  overflowMode=off
  Terminator : Terminator
  Transport Delay : TransportDelay  DelayTime=IMU.latency
  imu_out : Outport
  wires:
  Accelerometers/1(accels_out) -> Accels/1, Mux/2  "Alpha_0_raw"
  Gyroscopes/1(gyros_out) -> Mux/1  "Omega_0_raw"
  Bus Creator/1 -> imu_out/1
  Transport Delay/1 -> Downsample/1
  Mux/1 -> Transport Delay/1
  Scalar Quantizer Encoder/1 -> Terminator/1
  Downsample/1 -> Demux1/1
  Demux1/1 -> Scalar Quantizer Encoder/1
  Scalar Quantizer Encoder/2 -> Bus Creator/1  "Omega_0"
  Demux1/2 -> Bus Creator/2  "Alpha_0"

== system cm_test/CarMaker/VehicleControl/Sensors/Magnetometer ==
  Bus Creator : BusCreator  Inputs='hdg'  OutDataTypeStr=Bus: mag_bus  NonVirtualBus=on
  Downsample : DownSample  N=mag.K_dn
  Scope : Scope
      settings: SaveName=ScopeData18
  Scope1 : Scope
      settings: TimeRange=10  YMin=-0.5  YMax=3.5  SaveName=ScopeData19
  vehicle heading : CarMaker4SL/Read CM Dict  xname=Vhcl.Yaw  xsync=off
  mag_out : Outport
  wires:
  Bus Creator/1 -> mag_out/1
  vehicle heading/1 -> Scope/1, Downsample/1
  Downsample/1 -> Scope1/1, Bus Creator/1  "hdg"

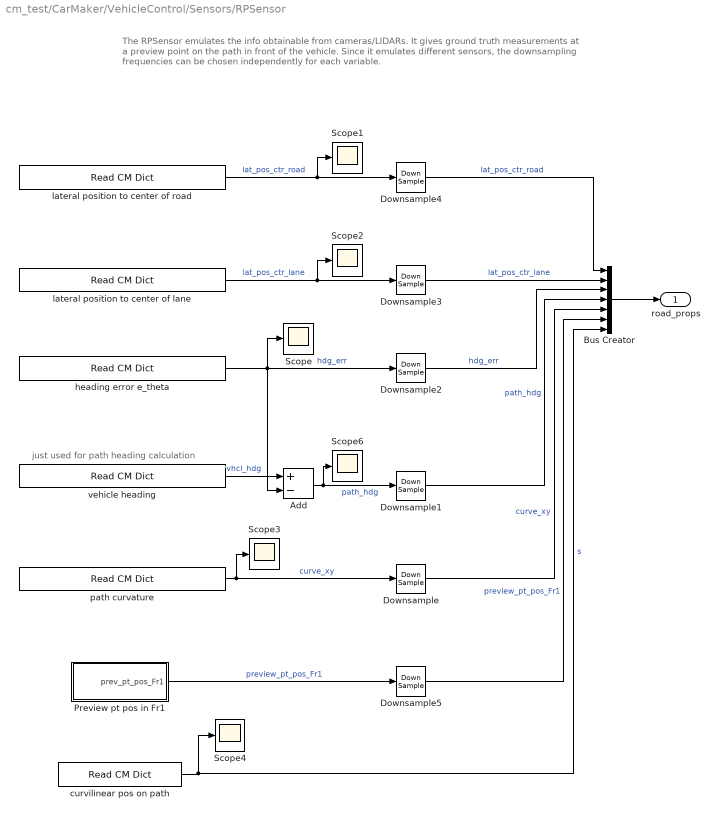
== system cm_test/CarMaker/VehicleControl/Sensors/RPSensor ==
  note: The RPSensor emulates the info obtainable from cameras/LIDARs.
      |
      | It gives ground truth measurements at a preview point on the path in front of the vehicle. Since it emulates different sensors, the downsampling frequencies can be chosen independently for each variable.
  note: just used for path heading calculation
  Add : Sum  Inputs=+-
  Bus Creator : BusCreator  Inputs='lat_pos_ctr_road','lat_pos_ctr_lane','hdg_err','path_hdg','curve_xy','preview_pt_pos_Fr1','s'  OutDataTypeStr=Bus: RPSensor_bus  NonVirtualBus=on
  Downsample{,1..5} (6 alike) : DownSample  N=1
  Preview pt pos in Fr1 : Subsystem
  Scope{,1..4,6} (6 alike) : Scope
      Scope settings: SaveName=ScopeData4  Decimation=10
      Scope1 settings: YMin=-1  YMax=10  SaveName=ScopeData3  Decimation=10
      Scope2 settings: SaveName=ScopeData5  Decimation=10
      Scope3 settings: SaveName=ScopeData12  Decimation=10
      Scope4 settings: SaveName=ScopeData22
      Scope6 settings: SaveName=ScopeData15  Decimation=10
  curvilinear pos on path : CarMaker4SL/Read CM Dict  xname=Vhcl.sRoad  xsync=off
  heading error e_theta : CarMaker4SL/Read CM Dict  xname=RPSensor.RP00.Path.DevAng  xsync=off
  lateral position to center of lane : CarMaker4SL/Read CM Dict  xname=RPSensor.RP00.Path.DevDist  xsync=off
  lateral position to center of road : CarMaker4SL/Read CM Dict  xname=RPSensor.RP00.Route.DevDist  xsync=off
  path curvature : CarMaker4SL/Read CM Dict  xname=RPSensor.RP00.Path.CurveXY  xsync=off
  vehicle heading : CarMaker4SL/Read CM Dict  xname=Vhcl.Yaw  xsync=off
  road_props : Outport
  wires:
  heading error e_theta/1 -> Scope/1, Downsample2/1, Add/2  "hdg_err"
  lateral position to center of road/1 -> Downsample4/1, Scope1/1  "lat_pos_ctr_road"
  lateral position to center of lane/1 -> Scope2/1, Downsample3/1  "lat_pos_ctr_lane"
  Bus Creator/1 -> road_props/1
  path curvature/1 -> Downsample/1, Scope3/1  "curve_xy"
  vehicle heading/1 -> Add/1  "vhcl_hdg"
  Add/1 -> Scope6/1, Downsample1/1  "path_hdg"
  Preview pt pos in Fr1/1(prev_pt_pos_Fr1) -> Downsample5/1  "preview_pt_pos_Fr1"
  Downsample/1 -> Bus Creator/5  "curve_xy"
  Downsample1/1 -> Bus Creator/4  "path_hdg"
  Downsample2/1 -> Bus Creator/3  "hdg_err"
  Downsample3/1 -> Bus Creator/2  "lat_pos_ctr_lane"
  Downsample4/1 -> Bus Creator/1  "lat_pos_ctr_road"
  Downsample5/1 -> Bus Creator/6  "preview_pt_pos_Fr1"
  curvilinear pos on path/1 -> Bus Creator/7, Scope4/1  "s"

== system cm_test/CarMaker/VehicleControl/Sensors/Steering angle (rad) ==
  Bus Creator : BusCreator  Inputs='steer_angle_1','steer_angle_2','mean_angle'  OutDataTypeStr=Bus: SteerSensor_bus  NonVirtualBus=on
  Downsample : DownSample  N=steer_sensor.K_dn
  Downsample1 : DownSample  N=steer_sensor.K_dn
  Gain : Gain  Gain=low_ctr.st_angle_to_st_wheel
  Mean of 2 values : Subsystem
  Mux : Mux  Inputs=2
  Mux1 : Mux  Inputs=2
  Read steering angle front left : CarMaker4SL/Read CM Dict  xname=Car.CFL.rz  xsync=off
  Read steering angle front right : CarMaker4SL/Read CM Dict  xname=Car.CFR.rz  xsync=off
  Scalar Quantizer Encoder : dspquant2/Scalar Quantizer Encoder  paramSrc=Specify via dialog  partType=Bounded  BBoundary=steer_sensor.bnd_pts  UBoundary=[2:9]  SearchMethod=Linear  tieBreakRule=Choose the lower index  outQU=on  outQError=off  codebook=steer_sensor.bnd_pts(1:end-1)  outStatus=off  invalidin=Clip  idtype=int32  roundingMode=Nearest  overflowMode=off
  Scalar Quantizer Encoder1 : dspquant2/Scalar Quantizer Encoder  paramSrc=Specify via dialog  partType=Bounded  BBoundary=steer_sensor.bnd_pts  UBoundary=[2:9]  SearchMethod=Linear  tieBreakRule=Choose the lower index  outQU=on  outQError=off  codebook=steer_sensor.bnd_pts(1:end-1)  outStatus=off  invalidin=Clip  idtype=int32  roundingMode=Nearest  overflowMode=off
  Scope{,1..4} (5 alike) : Scope
      Scope settings: YMin=-0.06  YMax=0.02  SaveName=ScopeData9
      Scope1 settings: SaveName=ScopeData10
      Scope2 settings: SaveName=ScopeData11
      Scope3 settings: ShowLegends=on  YMax=4  SaveName=ScopeData14
      Scope4 settings: SaveName=ScopeData16
  Terminator : Terminator
  Terminator1 : Terminator
  angle at steering wheel : CarMaker4SL/Read CM Dict  xname=Steer.WhlAng  xsync=off
  steer angles : Outport
  wires:
  Read steering angle front right/1 -> Downsample/1  "raw_steer_angle_1"
  Read steering angle front left/1 -> Scope/1, Downsample1/1  "raw_steer_angle_2"
  Mux/1 -> Mean of 2 values/1(vec)
  Mean of 2 values/1(mean) -> Scope4/1, Gain/1, Bus Creator/3  "mean_angle"
  Bus Creator/1 -> steer angles/1
  Downsample1/1 -> Scope1/1, Scalar Quantizer Encoder/1
  Scalar Quantizer Encoder/2 -> Scope2/1, Mux/1, Bus Creator/2  "steer_angle_2"
  Scalar Quantizer Encoder/1 -> Terminator/1  "steer_angle_2"
  Downsample/1 -> Scalar Quantizer Encoder1/1  "steer_angle_1"
  Scalar Quantizer Encoder1/1 -> Terminator1/1
  Scalar Quantizer Encoder1/2 -> Mux/2, Bus Creator/1  "steer_angle_1"
  angle at steering wheel/1 -> Mux1/2  "st_wheel"
  Mux1/1 -> Scope3/1
  Gain/1 -> Mux1/1  "est_st_wheel"

== system cm_test/CarMaker/VehicleControl/Sensors/odometry ==
  Bus Creator : BusCreator  Commented=on  Inputs='steer_angle_1','steer_angle_2','mean_angle'  OutDataTypeStr=Bus: SteerSensor_bus  NonVirtualBus=on
  Bus Creator1 : BusCreator  Inputs=1  OutDataTypeStr=Bus: OdoSensors_bus  NonVirtualBus=on
  Downsample : DownSample  Commented=on  N=steer_sensor.K_dn
  Downsample1 : DownSample  Commented=on  N=steer_sensor.K_dn
  Downsample2 : DownSample  N=odo.K_dn
  Mean of 2 values : Subsystem  Commented=on
  Mux : Mux  Commented=on  Inputs=2
  Mux1 : Mux  Inputs=3
  Read steering angle front left : CarMaker4SL/Read CM Dict  Commented=on  xname=wheel_odo  xsync=off
  Read steering angle front right : CarMaker4SL/Read CM Dict  Commented=on  xname=wheel_odo  xsync=off
  Scalar Quantizer Encoder : dspquant2/Scalar Quantizer Encoder  Commented=on  paramSrc=Specify via dialog  partType=Bounded  BBoundary=steer_sensor.bnd_pts  UBoundary=[2:9]  SearchMethod=Linear  tieBreakRule=Choose the lower index  outQU=on  outQError=off  codebook=steer_sensor.bnd_pts(1:end-1)  outStatus=off  invalidin=Clip  idtype=int32  roundingMode=Nearest  overflowMode=off
  Scalar Quantizer Encoder1 : dspquant2/Scalar Quantizer Encoder  Commented=on  paramSrc=Specify via dialog  partType=Bounded  BBoundary=steer_sensor.bnd_pts  UBoundary=[2:9]  SearchMethod=Linear  tieBreakRule=Choose the lower index  outQU=on  outQError=off  codebook=steer_sensor.bnd_pts(1:end-1)  outStatus=off  invalidin=Clip  idtype=int32  roundingMode=Nearest  overflowMode=off
  Scalar Quantizer Encoder2 : dspquant2/Scalar Quantizer Encoder  paramSrc=Specify via dialog  partType=Unbounded  BBoundary=steer_sensor.bnd_pts  UBoundary=odo.bnd_pts(1:end-1)  SearchMethod=Linear  tieBreakRule=Choose the lower index  outQU=on  outQError=off  codebook=odo.bnd_pts-0.05  outStatus=off  invalidin=Clip  idtype=int32  roundingMode=Nearest  overflowMode=off
  Scope : Scope
      settings: YMin=-1  YMax=9  SaveName=ScopeData20
  Terminator : Terminator  Commented=on
  Terminator1 : Terminator  Commented=on
  Terminator2 : Terminator
  Terminator3 : Terminator  Commented=on
  motor odometry (gives translational speed) : CarMaker4SL/Read CM Dict  xname=Vhcl.PoI.vx_1  xsync=off
  odo_out : Outport
  wires:
  Read steering angle front right/1 -> Downsample/1  "raw_steer_angle_1"
  Read steering angle front left/1 -> Downsample1/1  "raw_steer_angle_2"
  Mux/1 -> Mean of 2 values/1(vec)
  Mean of 2 values/1(mean) -> Bus Creator/3  "mean_angle"
  Bus Creator/1 -> Terminator3/1
  Downsample1/1 -> Scalar Quantizer Encoder/1
  Scalar Quantizer Encoder/2 -> Mux/1, Bus Creator/2  "steer_angle_2"
  Scalar Quantizer Encoder/1 -> Terminator/1  "steer_angle_2"
  Downsample/1 -> Scalar Quantizer Encoder1/1  "steer_angle_1"
  Scalar Quantizer Encoder1/1 -> Terminator1/1
  Scalar Quantizer Encoder1/2 -> Mux/2, Bus Creator/1  "steer_angle_1"
  motor odometry (gives translational speed)/1 -> Mux1/1, Downsample2/1  "st_wheel"
  Downsample2/1 -> Mux1/2, Scalar Quantizer Encoder2/1
  Scalar Quantizer Encoder2/1 -> Terminator2/1
  Scalar Quantizer Encoder2/2 -> Mux1/3, Bus Creator1/1  "vel_from_motor"
  Mux1/1 -> Scope/1  "speed"
  Bus Creator1/1 -> odo_out/1

== system cm_test/CarMaker/IPG Vehicle/CarAndTrailer/CarAndTrailerUpd/CreateBus Brake.IF.In ==
  In : Inport
  BusCreator : BusCreator  Inputs=9
  Demux : Demux  Outputs=9
  Out : Outport
  wires:
  Demux/9 -> BusCreator/9  "Brake IF Trq_Reg RR"
  Demux/8 -> BusCreator/8  "Brake IF Trq_Reg RL"
  Demux/7 -> BusCreator/7  "Brake IF Trq_Reg FR"
  Demux/6 -> BusCreator/6  "Brake IF Trq_Reg FL"
  Demux/5 -> BusCreator/5  "Brake IF Trq_Reg_max RR"
  Demux/4 -> BusCreator/4  "Brake IF Trq_Reg_max RL"
  Demux/3 -> BusCreator/3  "Brake IF Trq_Reg_max FR"
  Demux/2 -> BusCreator/2  "Brake IF Trq_Reg_max FL"
  Demux/1 -> BusCreator/1  "Brake IF T_env"
  BusCreator/1 -> Out/1
  In/1 -> Demux/1
